simulink model "PIDModel"  (R2021b)
settings: Solver=VariableStepAuto  StartTime=0.0  StopTime=10.0  RelTol=1e-3
settings Model: Creator=Lenovo  LastModifiedBy=Lenovo

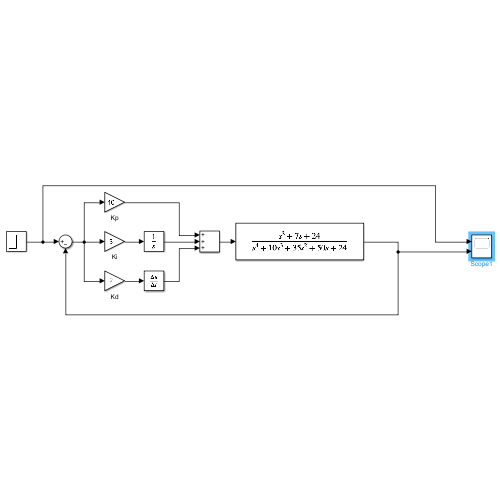
[thumbnail: Simulink's stored preview of the top-level diagram]
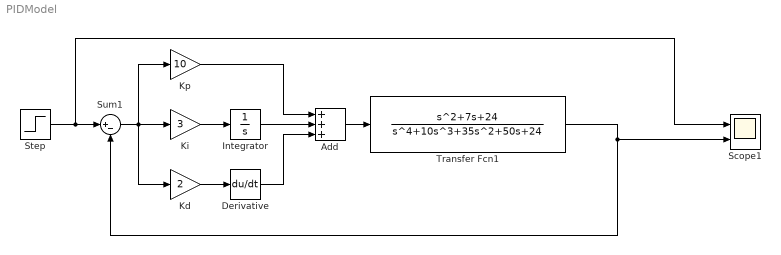
== system PIDModel ==
  Add : Sum  Inputs=+++
  Derivative : Derivative
  Integrator : Integrator
  Kd : Gain  Gain=2
  Ki : Gain  Gain=3
  Kp : Gain  Gain=10
  Scope1 : Scope  NumInputPorts=2
  Step : Step  Time=0  SampleTime=0
  Sum1 : Sum  Inputs=|+-
  Transfer Fcn1 : TransferFcn  Numerator=[1,7,24]  Denominator=[1,10,35,50,24]
  wires:
  Transfer Fcn1/1 -> Sum1/2, Scope1/2
  Ki/1 -> Integrator/1
  Kd/1 -> Derivative/1
  Integrator/1 -> Add/2
  Derivative/1 -> Add/3
  Kp/1 -> Add/1
  Sum1/1 -> Ki/1, Kd/1, Kp/1
  Add/1 -> Transfer Fcn1/1
  Step/1 -> Scope1/1, Sum1/1
